simulink model "SingalStable01"  (Simulink 8.1)
settings: Solver=ode45  StartTime=1  StopTime=2  MaxStep=0.000001  RelTol=1e-3
libraries: dsparch4 x3, commsynccomp2 x1, simulink x1
settings Model: Creator=my88899  LastModifiedBy=my88899
settings SolverCC: ConsecutiveZCsStepRelTol=20*128*eps
settings DataIOCC: SignalLoggingSaveFormat=Dataset
settings OptimizationCC: ExpressionDepthLimit=128
settings DebuggingCC: FcnCallInpInsideContextMsg=EnableAllAsError
settings GRTTargetCC: CombineOutputUpdateFcns=on  GRTInterface=off

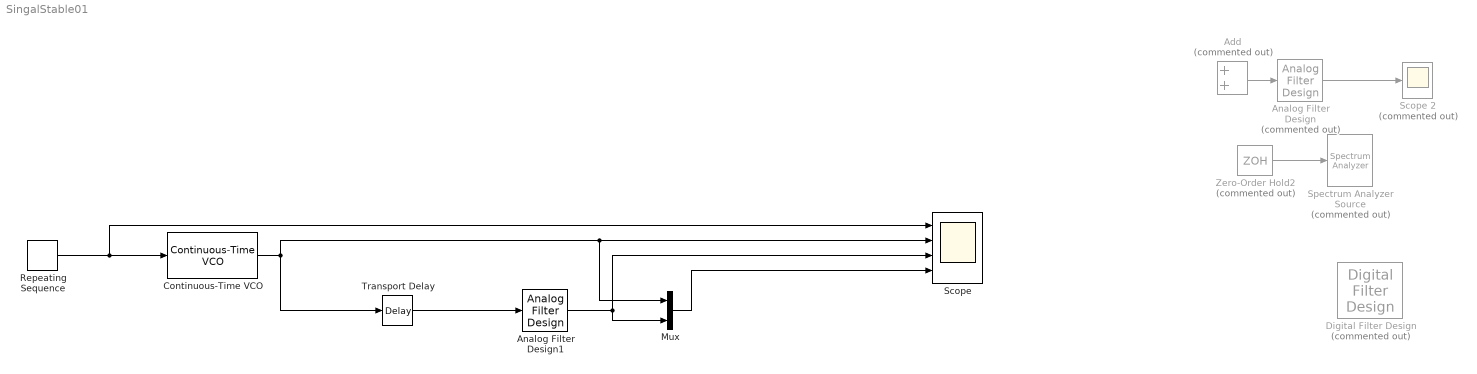
== system SingalStable01 ==
  Add : Sum  Commented=on
  Analog Filter Design : dsparch4/Analog Filter Design  Commented=on  method=Butterworth  filttype=Lowpass  N=12  Wlo=2*3.14*40000  Whi=80  Rp=2  Rs=40
  Analog Filter Design1 : dsparch4/Analog Filter Design  method=Butterworth  filttype=Lowpass  N=12  Wlo=2*3.14*40000  Whi=80  Rp=2  Rs=40
  Continuous-Time VCO : commsynccomp2/Continuous-Time VCO  Ac=5  Fc=100  Kc=10000  Ph=0
  Digital Filter Design : dsparch4/Digital Filter Design  Commented=on  mwdsp_browser_bugfix_var=off
  Mux : Mux  Inputs=2
  Repeating Sequence : simulink/Sources/Repeating Sequence  rep_seq_t=[0 2]  rep_seq_y=[0 4]
  Scope : Scope  NumInputPorts=4
      settings: TimeRange=0.1038961038961048  YMin=3.05~-5~-5~-5  YMax=3.5~5~5~5  MaxDataPoints=4000000
  "Scope 2 " : Scope  Commented=on
      settings: TimeRange=0.1038961038961048  YMin=-15  YMax=15  MaxDataPoints=10000001
  "Spectrum Analyzer Source " : SpectrumAnalyzer  Commented=on
      settings: CopyFcn=scopeextensions.ScopeBlock.callback(gcbh, 'onBlockCopy', gcbh);  DeleteFcn=scopeextensions.ScopeBlock.callback(gcbh, 'onBlockDelete');  PreSaveFcn=scopeextensions.ScopeBlock.callback(gcbh, 'onModelSave');  NameChangeFcn=scopeextensions.ScopeBlock.callback(gcbh, 'onBlockRename');  CloseFcn=scopeextensions.ScopeBlock.callback(gcbh, 'onBlockClose');  PreDeleteFcn=scopeextensions.ScopeBlock.callback(gcbh, 'onBlockPreDelete');
  Transport Delay : TransportDelay  DelayTime=0.3  BufferSize=400000
  Zero-Order Hold2 : ZeroOrderHold  Commented=on  SampleTime=0.001
  wires:
  Repeating Sequence/1 -> Scope/1, Continuous-Time VCO/1
  Zero-Order Hold2/1 -> "Spectrum Analyzer Source "/1
  Continuous-Time VCO/1 -> Transport Delay/1, Scope/2, Mux/1
  Transport Delay/1 -> Analog Filter Design1/1
  Add/1 -> Analog Filter Design/1
  Mux/1 -> Scope/4
  Analog Filter Design/1 -> "Scope 2 "/1
  Analog Filter Design1/1 -> Scope/3, Mux/2
